simulink model "platoon3"  (R2018b)
settings: Solver=FixedStepAuto  StartTime=0.0  StopTime=10.0  FixedStep=0.05  RelTol=1e-3  EnableMultiTasking=on
settings Model: Creator=Xiaodong  LastModifiedBy=Xiaodong
settings SolverCC: AutoInsertRateTranBlk=on
settings DataIOCC: LimitDataPoints=on
settings OptimizationCC: LifeSpan=inf
settings DebuggingCC: AllowSymbolicDim=off  SFUnexpectedBacktrackingDiag=warning  SFNoUnconditionalDefaultTransitionDiag=warning  SFExecutionAtInitializationDiag=none
settings SFSimCC: SimUseLocalCustomCode=off
settings RTWCC: RTWUseLocalCustomCode=off
settings CodeAppCC: StateflowObjectComments=on
settings GRTTargetCC: TargetLangStandard=C89/C90 (ANSI)  GeneratePreprocessorConditionals=Disable all
settings ConfigComp: CovMetricSettings=dw  CovHtmlReporting=on  CovSaveCumulativeToWorkspaceVar=on  CovSaveSingleToWorkspaceVar=on  CovShowResultsExplorer=off  CovExternalEMLEnable=off  CovSFcnEnable=off

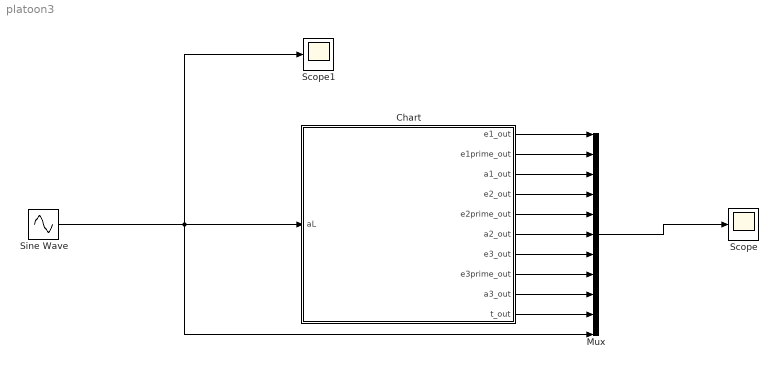
== system platoon3 ==
  Chart : Stateflow chart  TreatAsAtomicUnit=on
  Mux : Mux  Inputs=11
  Scope : Scope
  Scope1 : Scope
  Sine Wave : Sin  Amplitude=5  Bias=-4  Phase=0.785*0.5*5  SampleTime=0
  wires:
  Sine Wave/1 -> Mux/11, Scope1/1, Chart/1(aL)
  Chart/1(e1_out) -> Mux/1
  Chart/2(e1prime_out) -> Mux/2
  Chart/3(a1_out) -> Mux/3
  Chart/4(e2_out) -> Mux/4
  Chart/5(e2prime_out) -> Mux/5
  Chart/6(a2_out) -> Mux/6
  Chart/7(e3_out) -> Mux/7
  Chart/8(e3prime_out) -> Mux/8
  Chart/9(a3_out) -> Mux/9
  Mux/1 -> Scope/1
  Chart/10(t_out) -> Mux/10

== stateflow chart platoon3/Chart ==
  settings: updateMethod=CONTINUOUS
  state OK
    du:
    e1_dot = e1prime;
    e1prime_dot = -a1 + aL;
    a1_dot = 1.605*e1 + 4.868*e1prime - 3.5754*a1 - 0.8198*e2 + 0.427*e2prime - 0.045*a2 - 0.1942*e3 + 0.3626*e3prime - 0.0946*a3;
    e2_dot = e2prime;
    e2prime_dot= a1 - a2;
    a2_dot = 0.8718*e1 + 3.814*e1prime - 0.0754*a1 + 1.1936*e2 + 3.6258*e2prime - 3.2396*a2 - 0.595*e3 + 0.1294*e3prime - 0.0796*a3;
    e3_dot = e3prime;
    e3prime_dot = a2 - a3;
    a3_dot = 0.7132*e1 + 3.573*e1prime - 0.0964*a1 + 0.8472*e2 + 3.2568*e2prime - 0.0876*a2 + 1.2726*e3 + 3.072*e3prime - 3.1356*a3;
    t_dot = 1;
    e1_out = e1;
    e1prime_out = e1prime;
    a1_out = a1;
    e2_out = e2;
    e2prime_out = e2prime;
    a2_out = a2;
    e3_out = e3;
    e3prime_out = e3prime;
    a3_out = a3;
    t_out = t;
  state Corrupt
    du:
    e1_dot = e1prime;
    e1prime_dot = -a1 + aL ;
    a1_dot = 1.605*e1 + 4.868*e1prime - 3.5754*a1;
    e2_dot = e2prime ;
    e2prime_dot = a1 - a2 ;
    a2_dot = 1.1936*e2 + 3.6258*e2prime - 3.2396*a2 ;
    e3_dot = e3prime ;
    e3prime_dot = a2 - a3 ;
    a3_dot = 0.7132*e1 + 3.573*e1prime - 0.0964*a1 + 0.8472*e2 + 3.2568*e2prime - 0.0876*a2 + 1.2726*e3 + 3.072*e3prime - 3.1356*a3 ;
    t_dot = 1;
    e1_out = e1;
    e1prime_out = e1prime;
    a1_out = a1;
    e2_out = e2;
    e2prime_out = e2prime;
    a2_out = a2;
    e3_out = e3;
    e3prime_out = e3prime;
    a3_out = a3;
    t_out = t;
  (default) -> OK
  OK -> Corrupt : [t>=c2]{t=0;}
  Corrupt -> OK : [t>=c1]{t=0;}
  data: e1 local =0.9; e1prime local =0.9; a1 local =0.9; e2 local =0.9; e2prime local =0.9; a2 local =0.9; e3 local =0.9; e3prime local =0.9; a3 local =0.9; t local =0; c2 constant double =2; aL input; c1 constant double =2; e1_out output; e1prime_out output; a1_out output; e2_out output; e2prime_out output; a2_out output; e3_out output; e3prime_out output; a3_out output; t_out output
  data e1 settings: updateMethod=SF_CONTINUOUS_TIME_DATA
  data e1prime settings: updateMethod=SF_CONTINUOUS_TIME_DATA
  data a1 settings: updateMethod=SF_CONTINUOUS_TIME_DATA
  data e2 settings: updateMethod=SF_CONTINUOUS_TIME_DATA
  data e2prime settings: updateMethod=SF_CONTINUOUS_TIME_DATA
  data a2 settings: updateMethod=SF_CONTINUOUS_TIME_DATA
  data e3 settings: updateMethod=SF_CONTINUOUS_TIME_DATA
  data e3prime settings: updateMethod=SF_CONTINUOUS_TIME_DATA
  data a3 settings: updateMethod=SF_CONTINUOUS_TIME_DATA
  data t settings: updateMethod=SF_CONTINUOUS_TIME_DATA
